simulink model "PolePlacement"  (R2012b)
settings: Solver=ode5  StartTime=0.0  StopTime=10.0  FixedStep=.001  RelTol=1e-3
values from neighbouring files (symbols this model uses):
  B = [0; (I+m*L^2)/alpha; 0; m*L/alpha]    [Nonlinear_Inverted_Pendulum_Modern_m.m]    (also in PolePlacement_m.m = 0.1)
  comp2Den = conv([1 0],[1 100])    [PolePlacement_m.m]
  comp2Num = conv([1 10+1i*10],[1 10-1i*10])    [PolePlacement_m.m]
  g = 9.8    [Nonlinear_Inverted_Pendulum_Modern_m.m]    (also in PolePlacement_m.m)
  I = 0.006    [Nonlinear_Inverted_Pendulum_Modern_m.m]    (also in PolePlacement_m.m)
  K = place(A,B,POLES)    [Nonlinear_Inverted_Pendulum_Modern_m.m]    (also in PolePlacement_m.m = -500)
  l = 0.3    [PolePlacement_m.m]
  m = 0.2    [Nonlinear_Inverted_Pendulum_Modern_m.m]    (also in PolePlacement_m.m)
  M = 0.5    [Nonlinear_Inverted_Pendulum_Modern_m.m]    (also in PolePlacement_m.m)
  thetaInit = .1    (= 0.1)    [Nonlinear_Inverted_Pendulum_Modern_m.m]    (also in PolePlacement_m.m)
settings Model: Creator=Andrew  LastModifiedBy=Andrew

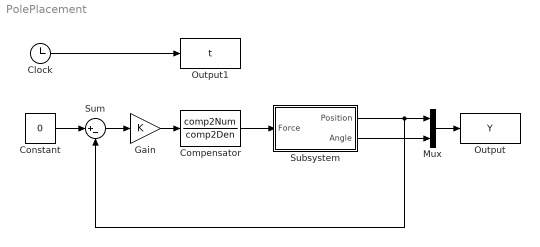
== system PolePlacement ==
  Clock : Clock
  Compensator : TransferFcn  Numerator=comp2Num  Denominator=comp2Den
  Constant : Constant  Value=0
  Gain : Gain  Gain=K
  Mux : Mux  Inputs=2
  Output : ToWorkspace  VariableName=Y  SampleTime=-1
  Output1 : ToWorkspace  VariableName=t  SampleTime=-1
  Subsystem : Subsystem
  Sum : Sum  Inputs=|+-
  wires:
  Sum/1 -> Gain/1
  Gain/1 -> Compensator/1
  Constant/1 -> Sum/1
  Clock/1 -> Output1/1
  Subsystem/1(Position) -> Sum/2, Mux/1
  Compensator/1 -> Subsystem/1(Force)
  Subsystem/2(Angle) -> Mux/2
  Mux/1 -> Output/1

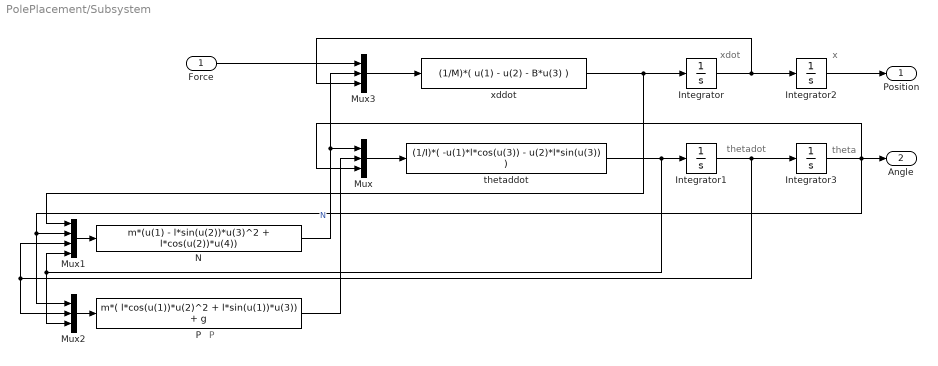
== system PolePlacement/Subsystem ==
  note: xdot
  note: x
  note: thetadot
  note: theta
  note: P
  Force : Inport
  Integrator : Integrator  ContinuousStateAttributes='xdot'
  Integrator1 : Integrator  ContinuousStateAttributes='thetadot'
  Integrator2 : Integrator  ContinuousStateAttributes='x'
  Integrator3 : Integrator  InitialCondition=thetaInit  ContinuousStateAttributes='theta'
  Mux : Mux  Inputs=3
  Mux1 : Mux
  Mux2 : Mux  Inputs=3
  Mux3 : Mux  Inputs=3
  N : Fcn  Expr=m*(u(1) - l*sin(u(2))*u(3)^2 + l*cos(u(2))*u(4))
  P : Fcn  Expr=m*( l*cos(u(1))*u(2)^2 + l*sin(u(1))*u(3)) + g
  thetaddot : Fcn  Expr=(1/I)*( -u(1)*l*cos(u(3)) - u(2)*l*sin(u(3)) )
  xddot : Fcn  Expr=(1/M)*( u(1) - u(2) - B*u(3) )
  Position : Outport
  Angle : Outport  Port=2
  wires:
  Integrator/1 -> Integrator2/1, Mux3/3
  Integrator1/1 -> Mux1/3, Mux2/2, Integrator3/1
  xddot/1 -> Integrator/1, Mux1/1
  thetaddot/1 -> Mux1/4, Mux2/3, Integrator1/1
  Mux/1 -> thetaddot/1
  Integrator2/1 -> Position/1
  Integrator3/1 -> Mux2/1, Mux1/2, Mux/3, Angle/1
  Mux1/1 -> N/1
  Mux3/1 -> xddot/1
  Force/1 -> Mux3/1
  N/1 -> Mux3/2, Mux/1  "N"
  Mux2/1 -> P/1
  P/1 -> Mux/2
